simulink model "TVModel_Simulation_21"  (R2021b)
settings: Solver=FixedStepDiscrete  StartTime=0.0  StopTime=250  FixedStep=0.02  MaxStep=0.01  RelTol=1e-3
undefined symbols (not defined in the file or in its folder): MB, TV, TV_OLD
libraries: simulink x22, simulink_extras x14, eeGeneralControl x13, slpidlib x8, fuzblock x4, controlLib x4, cstblocks x3, dspstat3 x2, eeSlidingModeController x1, sharedTrackingLibrary x1
(part 8 of 9)

== matlab function TVModel_Simulation_21/Subsystem/Subsystem1/Slip Control/Traction Control/ABS/Mu Linearization ==
  data: kappa input; mu0 output; mu1 output; Fz input; a0 output
function [mu0,mu1,a0] = fcn(kappa,Fz)

LMUX = 0.93;
J_wheel = 2e5/1e6;
rs = 0.235;
m = 270/4;
tau = 13.5;
dt = 0.02;

deltaKappa = 0.01;
kappa_plus = kappa + deltaKappa;

mu0 = muX(kappa,Fz,LMUX);
mu1 = (muX(kappa_plus,Fz,LMUX)-mu0)./(deltaKappa);

a0 = Fz./vx*mu1( (1-kappa)/m + rs^2/J_wheel );

end
function mu = muX(kappa,Fz,LMUX)
    mu = ((Fz.^2.*LMUX)./1.0e+4-Fz.*LMUX.*sin(atan((Fz.*5.946e-5-6.5736e-1).*(sign(Fz.*(-1.5696e-6)+kappa+6.665e-4).*5.242e-1+1.0).*(atan((Fz.*exp(Fz.*(-1.3455e-5)+1.3455e-2).*(Fz.*(3.0./2.0e+2)+6.77e+2./1.0e+1).*(Fz.*(-1.5696e-6)+kappa+6.665e-4).*(3.33e+2./4.0e+2))./(Fz.*LMUX.*2.5847808+1.0./1.0e+2))-(Fz.*exp(Fz.*(-1.3455e-5)+1.3455e-2).*(Fz.*(3.0./2.0e+2)+6.77e+2./1.0e+1).*(Fz.*(-1.5696e-6)+kappa+6.665e-4).*(3.33e+2./4.0e+2))./(Fz.*LMUX.*2.5847808+1.0./1.0e+2))-(Fz.*exp(Fz.*(-1.3455e-5)+1.3455e-2).*(Fz.*(3.0./2.0e+2)+6.77e+2./1.0e+1).*(Fz.*(-1.5696e-6)+kappa+6.665e-4).*(3.33e+2./4.0e+2))./(Fz.*LMUX.*2.5847808+1.0./1.0e+2)).*(1.68e+2./1.25e+2)).*1.9232)./Fz;
end

== stateflow chart TVModel_Simulation_21/Subsystem/Subsystem1/Slip Control/Traction Control/ABS/Subsystem/Chart ==
  state OFF
    en,du:
    TC_max = [21];
  state ON
    en,du:
    TC_max = T_ff ;
  state SWITCHING_FILTER
    en,du:
    TC_max = TC_filter_tau*TC_max;
  (default) -> OFF
  OFF -> ON : [epsilon == 1]
  SWITCHING_FILTER -> ON [order 2] : [ epsilon == 1]
  SWITCHING_FILTER -> OFF [order 1] : [count(in(SWITCHING_FILTER)) > TC_filter_time/ts]
  ON -> SWITCHING_FILTER : [epsilon == 0]
  data: T_ff input; TC_max output; ts constant double =TV.MPC.T; TC_filter_time constant double =TV.MPC.mz_filter_time; TC_filter_tau constant double =TV.MPC.mz_filter_tau; epsilon input

== matlab function TVModel_Simulation_21/Subsystem/Subsystem1/Torque Distribution/MPC/Useful Calculations/MATLAB Function2 ==
  data: omega input; y output; t input
function y = fcn(omega,t)

omega_FL = omega(1);
omega_FR = omega(2);
omega_RL = omega(3);
omega_RR = omega(4);

T_FL = t(1);
T_FR = t(2);
T_RL = t(3);
T_RR = t(4);

eta_FL = efficiency(omega_FL,T_FL) ;
eta_FR = efficiency(omega_FR,T_FR) ;
eta_RL = efficiency(omega_RL,T_RL) ;
eta_RR = efficiency(omega_RR,T_RR) ;

y = (omega_FL*T_FL/eta_FL + omega_FR*T_FR/eta_FR + omega_RL*T_RL/eta_RL + omega_RR*T_RR/eta_RR);

end

function eta = efficiency(Omega,T)

x = T;
y = Omega; % Omega rad/s to motor

p00 =      0.7189;
p10 =     0.06443;
p01 =   0.0001287;
p20 =     -0.0128;
p11 =   9.544e-05;
p02 =  -8.738e-07;
p30 =   0.0009902;
p21 =  -6.784e-06;
p12 =  -2.146e-08;
p03 =   8.018e-10;
p40 =  -3.737e-05;
p31 =   3.242e-07;
p22 =  -4.019e-10;
p13 =   9.786e-12;
p04 =   -3.44e-13;
p50 =   5.334e-07;
p41 =  -5.236e-09;
p32 =  -4.411e-14;
p23 =   1.035e-13;
p14 =  -1.745e-15;
p05 =   5.581e-17;

eta = p00 + p10*x + p01*y + p20*x^2 + p11*x*y + p02*y^2 + p30*x^3 + p21*x^2*y ...
      + p12*x*y^2 + p03*y^3 + p40*x^4 + p31*x^3*y + p22*x^2*y^2 ...
      + p13*x*y^3 + p04*y^4 + p50*x^5 + p41*x^4*y + p32*x^3*y^2 ...
      + p23*x^2*y^3 + p14*x*y^4 + p05*y^5;

end

== stateflow chart TVModel_Simulation_21/Subsystem/Subsystem1/Slip Control/Traction Control/Slip Control/ABS/Activation logic ==
  state TS_ON
    state ABS_OFF
      en,du:
      T_min(1:4) = -T_limit(1:4);
    state ABS_ON
      state FL [parallel]
        settings: executionOrder=1
        state ABS_ACTIVE
          en:
          T_min(1) = T_actual(1);
          du:
          T_min(1) = Tmin_PI(1);
        state ABS_INACTIVE
          en,du:
          T_min(1) = -T_limit(1);
        (default) -> TS_ON.ABS_ON.FL.ABS_INACTIVE
        TS_ON.ABS_ON.FL.ABS_INACTIVE -> TS_ON.ABS_ON.FL.ABS_ACTIVE : [eps(1) <= (epsTarget(1) - slipNoise) && T_actual(1)<0]
        TS_ON.ABS_ON.FL.ABS_ACTIVE -> TS_ON.ABS_ON.FL.ABS_INACTIVE : [T_actual(1) > slipDeactPerc*Tmin_old(1)]
      state FR [parallel]
        settings: executionOrder=2
        state ABS_ACTIVE
          en:
          T_min(2) = T_actual(2);
          du:
          T_min(2) = Tmin_PI(2);
        state ABS_INACTIVE
          en,du:
          T_min(2) = -T_limit(2);
        (default) -> TS_ON.ABS_ON.FR.ABS_INACTIVE
        TS_ON.ABS_ON.FR.ABS_INACTIVE -> TS_ON.ABS_ON.FR.ABS_ACTIVE : [eps(2) <= (epsTarget(2) - slipNoise) && T_actual(2)<0]
        TS_ON.ABS_ON.FR.ABS_ACTIVE -> TS_ON.ABS_ON.FR.ABS_INACTIVE : [T_actual(2) > slipDeactPerc*Tmin_old(2) ]
      state RL [parallel]
        settings: executionOrder=3
        state ABS_ACTIVE
          en:
          T_min(3) = T_actual(3);
          du:
          T_min(3) = Tmin_PI(3);
        state ABS_INACTIVE
          en,du:
          T_min(3) = -T_limit(3);
        (default) -> TS_ON.ABS_ON.RL.ABS_INACTIVE
        TS_ON.ABS_ON.RL.ABS_INACTIVE -> TS_ON.ABS_ON.RL.ABS_ACTIVE : [eps(3) <= (epsTarget(3) - slipNoise) && T_actual(3)<0]
        TS_ON.ABS_ON.RL.ABS_ACTIVE -> TS_ON.ABS_ON.RL.ABS_INACTIVE : [T_actual(3) > slipDeactPerc*Tmin_old(3)]
      state RR [parallel]
        settings: executionOrder=4
        state ABS_ACTIVE
          en:
          T_min(4) = T_actual(4);
          du:
          T_min(4) = Tmin_PI(4);
        state ABS_INACTIVE
          en,du:
          T_min(4) = -T_limit(4);
        (default) -> TS_ON.ABS_ON.RR.ABS_INACTIVE
        TS_ON.ABS_ON.RR.ABS_INACTIVE -> TS_ON.ABS_ON.RR.ABS_ACTIVE : [eps(4) <= (epsTarget(4) - slipNoise) && T_actual(4)<0]
        TS_ON.ABS_ON.RR.ABS_ACTIVE -> TS_ON.ABS_ON.RR.ABS_INACTIVE : [T_actual(4) > slipDeactPerc*Tmin_old(4)]
    (default) -> ABS_OFF
    ABS_ON -> ABS_OFF : [TC_flag == 0]
    ABS_OFF -> ABS_ON : [TC_flag == 1]
  state TS_OFF
    en:
    T_min(1:4) =zeros(4,1);
  (default) -> TS_OFF
  TS_OFF -> TS_ON : [RTD_flag == 1]
  TS_ON -> TS_OFF : [RTD_flag == 0]
  data: Tmin_PI input size=4; epsTarget input size=4; eps input size=4; T_actual input size=4 =zeros(4,1); T_min output size=4 =zeros(4,1); T_limit input size=4; TC_flag input size=1; Tmin_old input size=4; slipNoise input double =LV.SLIP.; slipDeactPerc input; RTD_flag input

== matlab function TVModel_Simulation_21/Subsystem/Subsystem1/Slip Control/Traction Control/Slip Control/Slip computation/MATLAB Function2 ==
  data: Vx input; V_FL output; Vy input; phi_dot input; delta_L input; V_FR output; V_RL output; V_RR output; alpha_FL output; alpha_FR output; alpha_RL output; alpha_RR output; delta_R input; a input; b input; t input; Vx_min input
function [V_FL,V_FR,V_RL,V_RR,alpha_FL,alpha_FR,alpha_RL,alpha_RR]= fcn(Vx,Vy,phi_dot, delta_L,delta_R,a,b,t,Vx_min)
   
    vx_max_den = max(Vx,Vx_min);

    V_FL = (Vx-(t/2)*phi_dot)*cos(delta_L)+(Vy+a*phi_dot)*sin(delta_L);
    alpha_FL = atan((Vy+a*phi_dot)/(vx_max_den -(t/2)*phi_dot))-delta_L;

    V_FR = (Vx+(t/2)*phi_dot)*cos(delta_R)+(Vy+a*phi_dot)*sin(delta_R);
    alpha_FR = atan((Vy+a*phi_dot)/(vx_max_den + (t/2)*phi_dot))-delta_R;

    V_RL = (((Vx-(t/2)*phi_dot)^2)+((Vy-b*phi_dot)^2))^(1/2);
    alpha_RL = atan((Vy-b*phi_dot)/(vx_max_den -(t/2)*phi_dot));

    V_RR = (((Vx+(t/2)*phi_dot)^2)+((Vy-b*phi_dot)^2))^(1/2);
    alpha_RR = atan((Vy-b*phi_dot)/(vx_max_den + (t/2)*phi_dot));
         
end

== stateflow chart TVModel_Simulation_21/Subsystem/Subsystem1/Slip Control/Traction Control/Slip Control/TC/Activation logic ==
  state TS_ON
    state TC_OFF
      en:TC_Active=uint8(ones(4,1));
      en,du:
      T_max(1:4) = T_limit(1:4);
    state TC_ON
      state FL [parallel]
        settings: executionOrder=1
        state TC_ACTIVE
          en:
          TC_Active(1)=uint8(2);
          T_max(1) = abs(T_actual(1));
          du:
          T_max(1) = Tmax_PI(1);
        state TC_INACTIVE
          en:
          TC_Active(1)=uint8(1);
          T_max(1) = T_limit(1);
          du:
          T_max(1) = T_limit(1);
        (default) -> TS_ON.TC_ON.FL.TC_INACTIVE
        TS_ON.TC_ON.FL.TC_INACTIVE -> TS_ON.TC_ON.FL.TC_ACTIVE : [eps(1) >= epsTarget(1) + slipNoise]
        TS_ON.TC_ON.FL.TC_ACTIVE -> TS_ON.TC_ON.FL.TC_INACTIVE : [T_actual(1) < slipDeactPerc*Tmax_old(1)]
      state FR [parallel]
        settings: executionOrder=2
        state TC_ACTIVE
          en:
          TC_Active(2)=uint8(2);
          T_max(2) = abs(T_actual(2));
          du:
          T_max(2) = Tmax_PI(2);
        state TC_INACTIVE
          en:
          TC_Active(2)=uint8(1);
          T_max(2) = T_limit(2);
          du:
          T_max(2) = T_limit(2);
        (default) -> TS_ON.TC_ON.FR.TC_INACTIVE
        TS_ON.TC_ON.FR.TC_INACTIVE -> TS_ON.TC_ON.FR.TC_ACTIVE : [eps(2) >= epsTarget(2) + slipNoise]
        TS_ON.TC_ON.FR.TC_ACTIVE -> TS_ON.TC_ON.FR.TC_INACTIVE : [T_actual(2) < slipDeactPerc*Tmax_old(2) ]
      state RL [parallel]
        settings: executionOrder=3
        state TC_ACTIVE
          en:
          TC_Active(3)=uint8(2);
          T_max(3) = abs(T_actual(3));
          du:
          T_max(3) = Tmax_PI(3);
        state TC_INACTIVE
          en:
          TC_Active(3)=uint8(1);
          T_max(3) = T_limit(3);
          du:
          T_max(3) = T_limit(3);
        (default) -> TS_ON.TC_ON.RL.TC_INACTIVE
        TS_ON.TC_ON.RL.TC_INACTIVE -> TS_ON.TC_ON.RL.TC_ACTIVE : [eps(3) >= epsTarget(3) + slipNoise]
        TS_ON.TC_ON.RL.TC_ACTIVE -> TS_ON.TC_ON.RL.TC_INACTIVE : [T_actual(3) < slipDeactPerc*Tmax_old(3)]
      state RR [parallel]
        settings: executionOrder=4
        state TC_ACTIVE
          en:
          TC_Active(4)=uint8(2);
          T_max(4) = abs(T_actual(4));
          du:
          T_max(4) = Tmax_PI(4);
        state TC_INACTIVE
          en:
          TC_Active(4)=uint8(1);
          T_max(4) = T_limit(4);
          du:
          T_max(4) = T_limit(4);
        (default) -> TS_ON.TC_ON.RR.TC_INACTIVE
        TS_ON.TC_ON.RR.TC_INACTIVE -> TS_ON.TC_ON.RR.TC_ACTIVE : [eps(4) >= epsTarget(4) + slipNoise]
        TS_ON.TC_ON.RR.TC_ACTIVE -> TS_ON.TC_ON.RR.TC_INACTIVE : [T_actual(4) < slipDeactPerc*Tmax_old(4)]
    (default) -> TC_OFF
    TC_ON -> TC_OFF : [TC_flag == 0]
    TC_OFF -> TC_ON : [TC_flag == 1]
  state TS_OFF
    en:
    T_max(1:4) = zeros(4,1);
  (default) -> TS_OFF
  TS_OFF -> TS_ON : [RTD_flag == 1]
  TS_ON -> TS_OFF : [RTD_flag == 0]
  data: Tmax_PI input size=4; epsTarget input size=4; eps input size=4; T_actual input size=4 =zeros(4,1); T_max output size=4 =zeros(4,1); T_limit input size=4; TC_flag input size=1; Tmax_old input size=4; slipNoise input double =LV.slipNoise; slipDeactPerc input; RTD_flag input; TC_Active output uint8 size=4

== matlab function TVModel_Simulation_21/Subsystem/Subsystem1/Slip Control/Traction Control/Slip Control/slip ratio/MATLAB Function ==
  data: vx_wheels input size=4; k output size=4; wR input size=4; vx_min input
function k = slipRatio(vx_wheels,wR,vx_min)

k = zeros(4,1);

for i = 1:4
   k(i) = (wR(i) - vx_wheels(i))/max([vx_wheels(i), wR(i), vx_min]);
end

end

== matlab function TVModel_Simulation_21/Subsystem/Subsystem1/Torque Distribution/MPC/Mz Generation/MATLAB Function3 ==
  data: ubx input; lbx input; Mzlim output; delta input
function Mzlim = fcn(ubx,lbx,delta)
tf = 1.27;
tr = 1.27;
a = 0.765;

delta_l = delta(1);
delta_r = delta(2);

T_FL_max = ubx(1);
T_FR_min = lbx(2);
T_RL_max = ubx(3);
T_RR_min = lbx(4);

Mzlim = +(a.*sin(delta_l)-tf/2.*cos(delta_l))*T_FL_max +(a.*sin(delta_r)+tf/2*cos(delta_r))*T_FR_min -tr/2*T_RL_max +tr/2*T_RR_min;

== matlab function TVModel_Simulation_21/Subsystem/Subsystem1/Torque Distribution/MPC/Mz Generation/MATLAB Function4 ==
  data: ubx input; lbx input; Mzlim output; delta input
function Mzlim = fcn(ubx,lbx,delta)
tf = 1.27;
tr = 1.27;
a = 0.765;

delta_l = delta(1);
delta_r = delta(2);

T_FL_min = lbx(1);
T_FR_max = ubx(2);
T_RL_min = lbx(3);
T_RR_max = ubx(4);

Mzlim = +(a.*sin(delta_l)-tf/2.*cos(delta_l))*T_FL_min +(a.*sin(delta_r)+tf/2*cos(delta_r))*T_FR_max -tr/2*T_RL_min +tr/2*T_RR_max;

== matlab function TVModel_Simulation_21/Subsystem/Subsystem1/Torque Distribution/MPC/Useful Calculations/MATLAB Function1 ==
  data: u input; deltag3 output; deltag4 output
function [deltag3,deltag4] = fcn(u)

deltag3 = u(2) - u(4);
deltag4 = u(1) - u(3);

== matlab function TVModel_Simulation_21/Subsystem/Subsystem1/Slip Control/Traction Control/TC/MATLAB Function ==
  data: u_max_old input; vx input; u output; Fz input; kappa input
function u = linear_mpc(u_max_old,vx,Fz,kappa)

LMU = 0.8;
rs = 0.235;
Iw = 2e5/1e6;
dt = 0.2;
tau = 13.5;
dt = 0.02;
g = 9.81;

B = rs^2/Iw/vx*dt;

u = zeros(4,1);
u(1) = tc(u_max_old(1),vx,Fz(1),kappa(1));
u(2) = tc(u_max_old(2),vx,Fz(2),kappa(2));
u(3) = tc(u_max_old(3),vx,Fz(3),kappa(3));
u(4) = tc(u_max_old(4),vx,Fz(4),kappa(4));

end
% Astar = (0.0148*cos(0.989*atan((atan(0.159/(635.0*kappa^2 + 1.0)^(1/2)) - 0.159/(635.0*kappa^2 + 1.0)^(1/2))*(2.08e-4*Fz + 0.117) - 0.159/(635.0*kappa^2 + 1.0)^(1/2)))*(1.0e-4*Fz^2*LMU - 1.92*Fz*LMU*sin(1.41*atan((4.17e-5*Fz - 0.46)*(0.524*sign(kappa - 1.57e-6*Fz + 6.66e-4) + 1.0)*(atan((0.7*Fz*exp(0.0135 - 1.35e-5*Fz)*(0.015*Fz + 67.7)*(kappa - 1.57e-6*Fz + 6.66e-4))/(2.71*Fz*LMU + 0.01)) - (0.7*Fz*exp(0.0135 - 1.35e-5*Fz)*(0.015*Fz + 67.7)*(kappa - 1.57e-6*Fz + 6.66e-4))/(2.71*Fz*LMU + 0.01)) - (0.7*Fz*exp(0.0135 - 1.35e-5*Fz)*(0.015*Fz + 67.7)*(kappa - 1.57e-6*Fz + 6.66e-4))/(2.71*Fz*LMU + 0.01)))))/(vx*cos(0.989*atan(0.159/(635.0*kappa^2 + 1.0)^(1/2) - 1.0*(atan(0.159/(635.0*kappa^2 + 1.0)^(1/2)) - 0.159/(635.0*kappa^2 + 1.0)^(1/2))*(2.08e-4*Fz + 0.117)))) + (0.989*sin(0.989*atan((atan(0.159/(635.0*kappa^2 + 1.0)^(1/2)) - 0.159/(635.0*kappa^2 + 1.0)^(1/2))*(2.08e-4*Fz + 0.117) - 0.159/(635.0*kappa^2 + 1.0)^(1/2)))*(1.0e-4*Fz^2*LMU - 1.92*Fz*LMU*sin(1.41*atan((4.17e-5*Fz - 0.46)*(0.524*sign(kappa - 1.57e-6*Fz + 6.66e-4) + 1.0)*(atan((0.7*Fz*exp(0.0135 - 1.35e-5*Fz)*(0.015*Fz + 67.7)*(kappa - 1.57e-6*Fz + 6.66e-4))/(2.71*Fz*LMU + 0.01)) - (0.7*Fz*exp(0.0135 - 1.35e-5*Fz)*(0.015*Fz + 67.7)*(kappa - 1.57e-6*Fz + 6.66e-4))/(2.71*Fz*LMU + 0.01)) - (0.7*Fz*exp(0.0135 - 1.35e-5*Fz)*(0.015*Fz + 67.7)*(kappa - 1.57e-6*Fz + 6.66e-4))/(2.71*Fz*LMU + 0.01))))*((2.08e-4*Fz + 0.117)*((101.0*kappa)/(635.0*kappa^2 + 1.0)^(3/2) - (101.0*kappa)/((635.0*kappa^2 + 1.0)^(3/2)*(0.0254/(635.0*kappa^2 + 1.0) + 1.0))) + (101.0*kappa)/(635.0*kappa^2 + 1.0)^(3/2))*(rs^2/Iw - 0.0148*kappa + 0.0148))/(vx*cos(0.989*atan(0.159/(635.0*kappa^2 + 1.0)^(1/2) - 1.0*(atan(0.159/(635.0*kappa^2 + 1.0)^(1/2)) - 0.159/(635.0*kappa^2 + 1.0)^(1/2))*(2.08e-4*Fz + 0.117)))*(((atan(0.159/(635.0*kappa^2 + 1.0)^(1/2)) - 0.159/(635.0*kappa^2 + 1.0)^(1/2))*(2.08e-4*Fz + 0.117) - 0.159/(635.0*kappa^2 + 1.0)^(1/2))^2 + 1.0)) + (0.989*cos(0.989*atan((atan(0.159/(635.0*kappa^2 + 1.0)^(1/2)) - 0.159/(635.0*kappa^2 + 1.0)^(1/2))*(2.08e-4*Fz + 0.117) - 0.159/(635.0*kappa^2 + 1.0)^(1/2)))*sin(0.989*atan(0.159/(635.0*kappa^2 + 1.0)^(1/2) - 1.0*(atan(0.159/(635.0*kappa^2 + 1.0)^(1/2)) - 0.159/(635.0*kappa^2 + 1.0)^(1/2))*(2.08e-4*Fz + 0.117)))*(1.0e-4*Fz^2*LMU - 1.92*Fz*LMU*sin(1.41*atan((4.17e-5*Fz - 0.46)*(0.524*sign(kappa - 1.57e-6*Fz + 6.66e-4) + 1.0)*(atan((0.7*Fz*exp(0.0135 - 1.35e-5*Fz)*(0.015*Fz + 67.7)*(kappa - 1.57e-6*Fz + 6.66e-4))/(2.71*Fz*LMU + 0.01)) - (0.7*Fz*exp(0.0135 - 1.35e-5*Fz)*(0.015*Fz + 67.7)*(kappa - 1.57e-6*Fz + 6.66e-4))/(2.71*Fz*LMU + 0.01)) - (0.7*Fz*exp(0.0135 - 1.35e-5*Fz)*(0.015*Fz + 67.7)*(kappa - 1.57e-6*Fz + 6.66e-4))/(2.71*Fz*LMU + 0.01))))*((2.08e-4*Fz + 0.117)*((101.0*kappa)/(635.0*kappa^2 + 1.0)^(3/2) - (101.0*kappa)/((635.0*kappa^2 + 1.0)^(3/2)*(0.0253/(635.0*kappa^2 + 1.0) + 1.0))) + (101.0*kappa)/(635.0*kappa^2 + 1.0)^(3/2))*(rs^2/Iw - 0.0148*kappa + 0.0148))/(vx*cos(0.989*atan(0.159/(635.0*kappa^2 + 1.0)^(1/2) - 1.0*(atan(0.159/(635.0*kappa^2 + 1.0)^(1/2)) - 0.159/(635.0*kappa^2 + 1.0)^(1/2))*(2.08e-4*Fz + 0.117)))^2*((1.0*(atan(0.159/(635.0*kappa^2 + 1.0)^(1/2)) - 0.159/(635.0*kappa^2 + 1.0)^(1/2))*(2.08e-4*Fz + 0.117) - 0.159/(635.0*kappa^2 + 1.0)^(1/2))^2 + 1.0)) - (2.71*Fz*LMU*cos(1.41*atan((4.17e-5*Fz - 0.46)*(0.524*sign(kappa - 1.57e-6*Fz + 6.66e-4) + 1.0)*(atan((0.7*Fz*exp(0.0135 - 1.35e-5*Fz)*(0.015*Fz + 67.7)*(kappa - 1.57e-6*Fz + 6.66e-4))/(2.71*Fz*LMU + 0.01)) - (0.7*Fz*exp(0.0135 - 1.35e-5*Fz)*(0.015*Fz + 67.7)*(kappa - 1.57e-6*Fz + 6.66e-4))/(2.71*Fz*LMU + 0.01)) - (0.7*Fz*exp(0.0135 - 1.35e-5*Fz)*(0.015*Fz + 67.7)*(kappa - 1.57e-6*Fz + 6.66e-4))/(2.71*Fz*LMU + 0.01)))*cos(0.989*atan((atan(0.159/(635.0*kappa^2 + 1.0)^(1/2)) - 0.159/(635.0*kappa^2 + 1.0)^(1/2))*(2.08e-4*Fz + 0.117) - 0.159/(635.0*kappa^2 + 1.0)^(1/2)))*(((0.7*Fz*exp(0.0135 - 1.35e-5*Fz)*(0.015*Fz + 67.7))/(2.71*Fz*LMU + 0.01) - (0.7*Fz*exp(0.0135 - 1.35e-5*Fz)*(0.015*Fz + 67.7))/(((0.49*Fz^2*exp(0.027 - 2.7e-5*Fz)*(0.015*Fz + 67.7)^2*(kappa - 1.57e-6*Fz + 6.66e-4)^2)/(2.71*Fz*LMU + 0.01)^2 + 1.0)*(2.71*Fz*LMU + 0.01)))*(4.17e-5*Fz - 0.46)*(0.524*sign(kappa - 1.57e-6*Fz + 6.66e-4) + 1.0) - 1.05*dirac(kappa - 1.57e-6*Fz + 6.66e-4)*(4.17e-5*Fz - 0.46)*(atan((0.7*Fz*exp(0.0135 - 1.35e-5*Fz)*(0.015*Fz + 67.7)*(kappa - 1.57e-6*Fz + 6.66e-4))/(2.71*Fz*LMU + 0.01)) - (0.7*Fz*exp(0.0135 - 1.35e-5*Fz)*(0.015*Fz + 67.7)*(kappa - 1.57e-6*Fz + 6.66e-4))/(2.71*Fz*LMU + 0.01)) + (0.7*Fz*exp(0.0135 - 1.35e-5*Fz)*(0.015*Fz + 67.7))/(2.71*Fz*LMU + 0.01))*(rs^2/Iw - 0.0148*kappa + 0.0148))/(vx*cos(0.989*atan(0.159/(635.0*kappa^2 + 1.0)^(1/2) - 1.0*(atan(0.159/(635.0*kappa^2 + 1.0)^(1/2)) - 0.159/(635.0*kappa^2 + 1.0)^(1/2))*(2.08e-4*Fz + 0.117)))*(((4.17e-5*Fz - 0.46)*(0.524*sign(kappa - 1.57e-6*Fz + 6.66e-4) + 1.0)*(atan((0.7*Fz*exp(0.0135 - 1.35e-5*Fz)*(0.015*Fz + 67.7)*(kappa - 1.57e-6*Fz + 6.66e-4))/(2.71*Fz*LMU + 0.01)) - (0.7*Fz*exp(0.0135 - 1.35e-5*Fz)*(0.015*Fz + 67.7)*(kappa - 1.57e-6*Fz + 6.66e-4))/(2.71*Fz*LMU + 0.01)) - (0.7*Fz*exp(0.0135 - 1.35e-5*Fz)*(0.015*Fz + 67.7)*(kappa - 1.57e-6*Fz + 6.66e-4))/(2.71*Fz*LMU + 0.01))^2 + 1.0))
function u_ij = tc(u_max_old,vx,Fz,kappa)
fx = -(1.0*cos(0.989*atan((atan(0.159/(635.0*kappa^2 + 1.0)^(1/2)) - 0.159/(635.0*kappa^2 + 1.0)^(1/2))*(2.08e-4*Fz + 0.117) - 0.159/(635.0*kappa^2 + 1.0)^(1/2)))*(1.0e-4*Fz^2*LMU - 1.92*Fz*LMU*sin(1.41*atan((4.17e-5*Fz - 0.46)*(0.524*sign(kappa - 1.57e-6*Fz + 6.66e-4) + 1.0)*(atan((0.7*Fz*exp(0.0135 - 1.35e-5*Fz)*(0.015*Fz + 67.7)*(kappa - 1.57e-6*Fz + 6.66e-4))/(2.71*Fz*LMU + 0.01)) - (0.7*Fz*exp(0.0135 - 1.35e-5*Fz)*(0.015*Fz + 67.7)*(kappa - 1.57e-6*Fz + 6.66e-4))/(2.71*Fz*LMU + 0.01)) - (0.7*Fz*exp(0.0135 - 1.35e-5*Fz)*(0.015*Fz + 67.7)*(kappa - 1.57e-6*Fz + 6.66e-4))/(2.71*Fz*LMU + 0.01))))*(rs^2/Iw - 0.0148*kappa + 0.0148))/(vx*cos(0.989*atan((atan(0.159/(635.0*kappa^2 + 1.0)^(1/2)) - 0.159/(635.0*kappa^2 + 1.0)^(1/2))*(2.08e-4*Fz + 0.117) - 0.159/(635.0*kappa^2 + 1.0)^(1/2))));
delta_kappa = 0.001;
kappa_plus = kappa + delta_kappa;
fx_plus = -(1.0*cos(0.989*atan((atan(0.159/(635.0*kappa_plus^2 + 1.0)^(1/2)) - 0.159/(635.0*kappa_plus^2 + 1.0)^(1/2))*(2.08e-4*Fz + 0.117) - 0.159/(635.0*kappa_plus^2 + 1.0)^(1/2)))*(1.0e-4*Fz^2*LMU - 1.92*Fz*LMU*sin(1.41*atan((4.17e-5*Fz - 0.46)*(0.524*sign(kappa_plus - 1.57e-6*Fz + 6.66e-4) + 1.0)*(atan((0.7*Fz*exp(0.0135 - 1.35e-5*Fz)*(0.015*Fz + 67.7)*(kappa_plus - 1.57e-6*Fz + 6.66e-4))/(2.71*Fz*LMU + 0.01)) - (0.7*Fz*exp(0.0135 - 1.35e-5*Fz)*(0.015*Fz + 67.7)*(kappa_plus - 1.57e-6*Fz + 6.66e-4))/(2.71*Fz*LMU + 0.01)) - (0.7*Fz*exp(0.0135 - 1.35e-5*Fz)*(0.015*Fz + 67.7)*(kappa_plus - 1.57e-6*Fz + 6.66e-4))/(2.71*Fz*LMU + 0.01))))*(rs^2/Iw - 0.0148*kappa_plus + 0.0148))/(vx*cos(0.989*atan((atan(0.159/(635.0*kappa_plus^2 + 1.0)^(1/2)) - 0.159/(635.0*kappa_plus^2 + 1.0)^(1/2))*(2.08e-4*Fz + 0.117) - 0.159/(635.0*kappa_plus^2 + 1.0)^(1/2))));

Astar = (fx_plus - fx)/delta_kappa;

A = (1 + Astar*dt);

% ~~~~~~~~~~~~~~~~~~~~~~~~~~~~~~~~~~~~~~~~~~~~~~~~~~~~~~~~~~~~~~~~~~~~~~~ %
kappa_ref = 0.1;

% Q = 1e6;
Q = 5e5;
R = 0e-5;

u_ij = u_max_old + (B*Q*B + R)*( (Q*B)*kappa_ref - (A*Q*B)*kappa )/tau;
end

== matlab function TVModel_Simulation_21/Subsystem/Subsystem1/Slip Control/Traction Control/Subsystem2/MATLAB Function1 ==
  data: u_max_old input; vx input; u output; Fz input; kappa input
function u = linear_mpc(u_max_old,vx,Fz,kappa)

% Astar = (0.0148*cos(0.989*atan((atan(0.159/(635.0*kappa^2 + 1.0)^(1/2)) - 0.159/(635.0*kappa^2 + 1.0)^(1/2))*(2.08e-4*Fz + 0.117) - 0.159/(635.0*kappa^2 + 1.0)^(1/2)))*(1.0e-4*Fz^2*LMU - 1.92*Fz*LMU*sin(1.41*atan((4.17e-5*Fz - 0.46)*(0.524*sign(kappa - 1.57e-6*Fz + 6.66e-4) + 1.0)*(atan((0.7*Fz*exp(0.0135 - 1.35e-5*Fz)*(0.015*Fz + 67.7)*(kappa - 1.57e-6*Fz + 6.66e-4))/(2.71*Fz*LMU + 0.01)) - (0.7*Fz*exp(0.0135 - 1.35e-5*Fz)*(0.015*Fz + 67.7)*(kappa - 1.57e-6*Fz + 6.66e-4))/(2.71*Fz*LMU + 0.01)) - (0.7*Fz*exp(0.0135 - 1.35e-5*Fz)*(0.015*Fz + 67.7)*(kappa - 1.57e-6*Fz + 6.66e-4))/(2.71*Fz*LMU + 0.01)))))/(vx*cos(0.989*atan(0.159/(635.0*kappa^2 + 1.0)^(1/2) - 1.0*(atan(0.159/(635.0*kappa^2 + 1.0)^(1/2)) - 0.159/(635.0*kappa^2 + 1.0)^(1/2))*(2.08e-4*Fz + 0.117)))) + (0.989*sin(0.989*atan((atan(0.159/(635.0*kappa^2 + 1.0)^(1/2)) - 0.159/(635.0*kappa^2 + 1.0)^(1/2))*(2.08e-4*Fz + 0.117) - 0.159/(635.0*kappa^2 + 1.0)^(1/2)))*(1.0e-4*Fz^2*LMU - 1.92*Fz*LMU*sin(1.41*atan((4.17e-5*Fz - 0.46)*(0.524*sign(kappa - 1.57e-6*Fz + 6.66e-4) + 1.0)*(atan((0.7*Fz*exp(0.0135 - 1.35e-5*Fz)*(0.015*Fz + 67.7)*(kappa - 1.57e-6*Fz + 6.66e-4))/(2.71*Fz*LMU + 0.01)) - (0.7*Fz*exp(0.0135 - 1.35e-5*Fz)*(0.015*Fz + 67.7)*(kappa - 1.57e-6*Fz + 6.66e-4))/(2.71*Fz*LMU + 0.01)) - (0.7*Fz*exp(0.0135 - 1.35e-5*Fz)*(0.015*Fz + 67.7)*(kappa - 1.57e-6*Fz + 6.66e-4))/(2.71*Fz*LMU + 0.01))))*((2.08e-4*Fz + 0.117)*((101.0*kappa)/(635.0*kappa^2 + 1.0)^(3/2) - (101.0*kappa)/((635.0*kappa^2 + 1.0)^(3/2)*(0.0254/(635.0*kappa^2 + 1.0) + 1.0))) + (101.0*kappa)/(635.0*kappa^2 + 1.0)^(3/2))*(rs^2/Iw - 0.0148*kappa + 0.0148))/(vx*cos(0.989*atan(0.159/(635.0*kappa^2 + 1.0)^(1/2) - 1.0*(atan(0.159/(635.0*kappa^2 + 1.0)^(1/2)) - 0.159/(635.0*kappa^2 + 1.0)^(1/2))*(2.08e-4*Fz + 0.117)))*(((atan(0.159/(635.0*kappa^2 + 1.0)^(1/2)) - 0.159/(635.0*kappa^2 + 1.0)^(1/2))*(2.08e-4*Fz + 0.117) - 0.159/(635.0*kappa^2 + 1.0)^(1/2))^2 + 1.0)) + (0.989*cos(0.989*atan((atan(0.159/(635.0*kappa^2 + 1.0)^(1/2)) - 0.159/(635.0*kappa^2 + 1.0)^(1/2))*(2.08e-4*Fz + 0.117) - 0.159/(635.0*kappa^2 + 1.0)^(1/2)))*sin(0.989*atan(0.159/(635.0*kappa^2 + 1.0)^(1/2) - 1.0*(atan(0.159/(635.0*kappa^2 + 1.0)^(1/2)) - 0.159/(635.0*kappa^2 + 1.0)^(1/2))*(2.08e-4*Fz + 0.117)))*(1.0e-4*Fz^2*LMU - 1.92*Fz*LMU*sin(1.41*atan((4.17e-5*Fz - 0.46)*(0.524*sign(kappa - 1.57e-6*Fz + 6.66e-4) + 1.0)*(atan((0.7*Fz*exp(0.0135 - 1.35e-5*Fz)*(0.015*Fz + 67.7)*(kappa - 1.57e-6*Fz + 6.66e-4))/(2.71*Fz*LMU + 0.01)) - (0.7*Fz*exp(0.0135 - 1.35e-5*Fz)*(0.015*Fz + 67.7)*(kappa - 1.57e-6*Fz + 6.66e-4))/(2.71*Fz*LMU + 0.01)) - (0.7*Fz*exp(0.0135 - 1.35e-5*Fz)*(0.015*Fz + 67.7)*(kappa - 1.57e-6*Fz + 6.66e-4))/(2.71*Fz*LMU + 0.01))))*((2.08e-4*Fz + 0.117)*((101.0*kappa)/(635.0*kappa^2 + 1.0)^(3/2) - (101.0*kappa)/((635.0*kappa^2 + 1.0)^(3/2)*(0.0253/(635.0*kappa^2 + 1.0) + 1.0))) + (101.0*kappa)/(635.0*kappa^2 + 1.0)^(3/2))*(rs^2/Iw - 0.0148*kappa + 0.0148))/(vx*cos(0.989*atan(0.159/(635.0*kappa^2 + 1.0)^(1/2) - 1.0*(atan(0.159/(635.0*kappa^2 + 1.0)^(1/2)) - 0.159/(635.0*kappa^2 + 1.0)^(1/2))*(2.08e-4*Fz + 0.117)))^2*((1.0*(atan(0.159/(635.0*kappa^2 + 1.0)^(1/2)) - 0.159/(635.0*kappa^2 + 1.0)^(1/2))*(2.08e-4*Fz + 0.117) - 0.159/(635.0*kappa^2 + 1.0)^(1/2))^2 + 1.0)) - (2.71*Fz*LMU*cos(1.41*atan((4.17e-5*Fz - 0.46)*(0.524*sign(kappa - 1.57e-6*Fz + 6.66e-4) + 1.0)*(atan((0.7*Fz*exp(0.0135 - 1.35e-5*Fz)*(0.015*Fz + 67.7)*(kappa - 1.57e-6*Fz + 6.66e-4))/(2.71*Fz*LMU + 0.01)) - (0.7*Fz*exp(0.0135 - 1.35e-5*Fz)*(0.015*Fz + 67.7)*(kappa - 1.57e-6*Fz + 6.66e-4))/(2.71*Fz*LMU + 0.01)) - (0.7*Fz*exp(0.0135 - 1.35e-5*Fz)*(0.015*Fz + 67.7)*(kappa - 1.57e-6*Fz + 6.66e-4))/(2.71*Fz*LMU + 0.01)))*cos(0.989*atan((atan(0.159/(635.0*kappa^2 + 1.0)^(1/2)) - 0.159/(635.0*kappa^2 + 1.0)^(1/2))*(2.08e-4*Fz + 0.117) - 0.159/(635.0*kappa^2 + 1.0)^(1/2)))*(((0.7*Fz*exp(0.0135 - 1.35e-5*Fz)*(0.015*Fz + 67.7))/(2.71*Fz*LMU + 0.01) - (0.7*Fz*exp(0.0135 - 1.35e-5*Fz)*(0.015*Fz + 67.7))/(((0.49*Fz^2*exp(0.027 - 2.7e-5*Fz)*(0.015*Fz + 67.7)^2*(kappa - 1.57e-6*Fz + 6.66e-4)^2)/(2.71*Fz*LMU + 0.01)^2 + 1.0)*(2.71*Fz*LMU + 0.01)))*(4.17e-5*Fz - 0.46)*(0.524*sign(kappa - 1.57e-6*Fz + 6.66e-4) + 1.0) - 1.05*dirac(kappa - 1.57e-6*Fz + 6.66e-4)*(4.17e-5*Fz - 0.46)*(atan((0.7*Fz*exp(0.0135 - 1.35e-5*Fz)*(0.015*Fz + 67.7)*(kappa - 1.57e-6*Fz + 6.66e-4))/(2.71*Fz*LMU + 0.01)) - (0.7*Fz*exp(0.0135 - 1.35e-5*Fz)*(0.015*Fz + 67.7)*(kappa - 1.57e-6*Fz + 6.66e-4))/(2.71*Fz*LMU + 0.01)) + (0.7*Fz*exp(0.0135 - 1.35e-5*Fz)*(0.015*Fz + 67.7))/(2.71*Fz*LMU + 0.01))*(rs^2/Iw - 0.0148*kappa + 0.0148))/(vx*cos(0.989*atan(0.159/(635.0*kappa^2 + 1.0)^(1/2) - 1.0*(atan(0.159/(635.0*kappa^2 + 1.0)^(1/2)) - 0.159/(635.0*kappa^2 + 1.0)^(1/2))*(2.08e-4*Fz + 0.117)))*(((4.17e-5*Fz - 0.46)*(0.524*sign(kappa - 1.57e-6*Fz + 6.66e-4) + 1.0)*(atan((0.7*Fz*exp(0.0135 - 1.35e-5*Fz)*(0.015*Fz + 67.7)*(kappa - 1.57e-6*Fz + 6.66e-4))/(2.71*Fz*LMU + 0.01)) - (0.7*Fz*exp(0.0135 - 1.35e-5*Fz)*(0.015*Fz + 67.7)*(kappa - 1.57e-6*Fz + 6.66e-4))/(2.71*Fz*LMU + 0.01)) - (0.7*Fz*exp(0.0135 - 1.35e-5*Fz)*(0.015*Fz + 67.7)*(kappa - 1.57e-6*Fz + 6.66e-4))/(2.71*Fz*LMU + 0.01))^2 + 1.0))

LMU = 0.8;
rs = 0.235;
Iw = 2e5/1e6;
dt = 0.2;
tau = 13.5;
dt = 0.02;
g = 9.81;

B = rs^2/Iw/vx*dt;

fx = -(1.0*cos(0.989*atan((atan(0.159/(635.0*kappa^2 + 1.0)^(1/2)) - 0.159/(635.0*kappa^2 + 1.0)^(1/2))*(2.08e-4*Fz + 0.117) - 0.159/(635.0*kappa^2 + 1.0)^(1/2)))*(1.0e-4*Fz^2*LMU - 1.92*Fz*LMU*sin(1.41*atan((4.17e-5*Fz - 0.46)*(0.524*sign(kappa - 1.57e-6*Fz + 6.66e-4) + 1.0)*(atan((0.7*Fz*exp(0.0135 - 1.35e-5*Fz)*(0.015*Fz + 67.7)*(kappa - 1.57e-6*Fz + 6.66e-4))/(2.71*Fz*LMU + 0.01)) - (0.7*Fz*exp(0.0135 - 1.35e-5*Fz)*(0.015*Fz + 67.7)*(kappa - 1.57e-6*Fz + 6.66e-4))/(2.71*Fz*LMU + 0.01)) - (0.7*Fz*exp(0.0135 - 1.35e-5*Fz)*(0.015*Fz + 67.7)*(kappa - 1.57e-6*Fz + 6.66e-4))/(2.71*Fz*LMU + 0.01))))*(rs^2/Iw - 0.0148*kappa + 0.0148))/(vx*cos(0.989*atan((atan(0.159/(635.0*kappa^2 + 1.0)^(1/2)) - 0.159/(635.0*kappa^2 + 1.0)^(1/2))*(2.08e-4*Fz + 0.117) - 0.159/(635.0*kappa^2 + 1.0)^(1/2))));
delta_kappa = 0.001;
kappa_plus = kappa + delta_kappa;
fx_plus = -(1.0*cos(0.989*atan((atan(0.159/(635.0*kappa_plus^2 + 1.0)^(1/2)) - 0.159/(635.0*kappa_plus^2 + 1.0)^(1/2))*(2.08e-4*Fz + 0.117) - 0.159/(635.0*kappa_plus^2 + 1.0)^(1/2)))*(1.0e-4*Fz^2*LMU - 1.92*Fz*LMU*sin(1.41*atan((4.17e-5*Fz - 0.46)*(0.524*sign(kappa_plus - 1.57e-6*Fz + 6.66e-4) + 1.0)*(atan((0.7*Fz*exp(0.0135 - 1.35e-5*Fz)*(0.015*Fz + 67.7)*(kappa_plus - 1.57e-6*Fz + 6.66e-4))/(2.71*Fz*LMU + 0.01)) - (0.7*Fz*exp(0.0135 - 1.35e-5*Fz)*(0.015*Fz + 67.7)*(kappa_plus - 1.57e-6*Fz + 6.66e-4))/(2.71*Fz*LMU + 0.01)) - (0.7*Fz*exp(0.0135 - 1.35e-5*Fz)*(0.015*Fz + 67.7)*(kappa_plus - 1.57e-6*Fz + 6.66e-4))/(2.71*Fz*LMU + 0.01))))*(rs^2/Iw - 0.0148*kappa_plus + 0.0148))/(vx*cos(0.989*atan((atan(0.159/(635.0*kappa_plus^2 + 1.0)^(1/2)) - 0.159/(635.0*kappa_plus^2 + 1.0)^(1/2))*(2.08e-4*Fz + 0.117) - 0.159/(635.0*kappa_plus^2 + 1.0)^(1/2))));

Astar = (fx_plus - fx)/delta_kappa;

A = (1 + Astar*dt);

% ~~~~~~~~~~~~~~~~~~~~~~~~~~~~~~~~~~~~~~~~~~~~~~~~~~~~~~~~~~~~~~~~~~~~~~~ %
kappa_ref = 0.1;

% Q = 1e6;
Q = 1e3;
R = 0e-5;

u = u_max_old + (B*Q*B + R)*( (Q*B)*kappa_ref - (A*Q*B)*kappa )/tau;
end

== matlab function TVModel_Simulation_21/Subsystem/Subsystem1/Slip Control/Traction Control/Subsystem2/MATLAB Function2 ==
  data: u_max_old input; vx input; u output; Fz input; kappa input
function u = linear_mpc(u_max_old,vx,Fz,kappa)

% Astar = (0.0148*cos(0.989*atan((atan(0.159/(635.0*kappa^2 + 1.0)^(1/2)) - 0.159/(635.0*kappa^2 + 1.0)^(1/2))*(2.08e-4*Fz + 0.117) - 0.159/(635.0*kappa^2 + 1.0)^(1/2)))*(1.0e-4*Fz^2*LMU - 1.92*Fz*LMU*sin(1.41*atan((4.17e-5*Fz - 0.46)*(0.524*sign(kappa - 1.57e-6*Fz + 6.66e-4) + 1.0)*(atan((0.7*Fz*exp(0.0135 - 1.35e-5*Fz)*(0.015*Fz + 67.7)*(kappa - 1.57e-6*Fz + 6.66e-4))/(2.71*Fz*LMU + 0.01)) - (0.7*Fz*exp(0.0135 - 1.35e-5*Fz)*(0.015*Fz + 67.7)*(kappa - 1.57e-6*Fz + 6.66e-4))/(2.71*Fz*LMU + 0.01)) - (0.7*Fz*exp(0.0135 - 1.35e-5*Fz)*(0.015*Fz + 67.7)*(kappa - 1.57e-6*Fz + 6.66e-4))/(2.71*Fz*LMU + 0.01)))))/(vx*cos(0.989*atan(0.159/(635.0*kappa^2 + 1.0)^(1/2) - 1.0*(atan(0.159/(635.0*kappa^2 + 1.0)^(1/2)) - 0.159/(635.0*kappa^2 + 1.0)^(1/2))*(2.08e-4*Fz + 0.117)))) + (0.989*sin(0.989*atan((atan(0.159/(635.0*kappa^2 + 1.0)^(1/2)) - 0.159/(635.0*kappa^2 + 1.0)^(1/2))*(2.08e-4*Fz + 0.117) - 0.159/(635.0*kappa^2 + 1.0)^(1/2)))*(1.0e-4*Fz^2*LMU - 1.92*Fz*LMU*sin(1.41*atan((4.17e-5*Fz - 0.46)*(0.524*sign(kappa - 1.57e-6*Fz + 6.66e-4) + 1.0)*(atan((0.7*Fz*exp(0.0135 - 1.35e-5*Fz)*(0.015*Fz + 67.7)*(kappa - 1.57e-6*Fz + 6.66e-4))/(2.71*Fz*LMU + 0.01)) - (0.7*Fz*exp(0.0135 - 1.35e-5*Fz)*(0.015*Fz + 67.7)*(kappa - 1.57e-6*Fz + 6.66e-4))/(2.71*Fz*LMU + 0.01)) - (0.7*Fz*exp(0.0135 - 1.35e-5*Fz)*(0.015*Fz + 67.7)*(kappa - 1.57e-6*Fz + 6.66e-4))/(2.71*Fz*LMU + 0.01))))*((2.08e-4*Fz + 0.117)*((101.0*kappa)/(635.0*kappa^2 + 1.0)^(3/2) - (101.0*kappa)/((635.0*kappa^2 + 1.0)^(3/2)*(0.0254/(635.0*kappa^2 + 1.0) + 1.0))) + (101.0*kappa)/(635.0*kappa^2 + 1.0)^(3/2))*(rs^2/Iw - 0.0148*kappa + 0.0148))/(vx*cos(0.989*atan(0.159/(635.0*kappa^2 + 1.0)^(1/2) - 1.0*(atan(0.159/(635.0*kappa^2 + 1.0)^(1/2)) - 0.159/(635.0*kappa^2 + 1.0)^(1/2))*(2.08e-4*Fz + 0.117)))*(((atan(0.159/(635.0*kappa^2 + 1.0)^(1/2)) - 0.159/(635.0*kappa^2 + 1.0)^(1/2))*(2.08e-4*Fz + 0.117) - 0.159/(635.0*kappa^2 + 1.0)^(1/2))^2 + 1.0)) + (0.989*cos(0.989*atan((atan(0.159/(635.0*kappa^2 + 1.0)^(1/2)) - 0.159/(635.0*kappa^2 + 1.0)^(1/2))*(2.08e-4*Fz + 0.117) - 0.159/(635.0*kappa^2 + 1.0)^(1/2)))*sin(0.989*atan(0.159/(635.0*kappa^2 + 1.0)^(1/2) - 1.0*(atan(0.159/(635.0*kappa^2 + 1.0)^(1/2)) - 0.159/(635.0*kappa^2 + 1.0)^(1/2))*(2.08e-4*Fz + 0.117)))*(1.0e-4*Fz^2*LMU - 1.92*Fz*LMU*sin(1.41*atan((4.17e-5*Fz - 0.46)*(0.524*sign(kappa - 1.57e-6*Fz + 6.66e-4) + 1.0)*(atan((0.7*Fz*exp(0.0135 - 1.35e-5*Fz)*(0.015*Fz + 67.7)*(kappa - 1.57e-6*Fz + 6.66e-4))/(2.71*Fz*LMU + 0.01)) - (0.7*Fz*exp(0.0135 - 1.35e-5*Fz)*(0.015*Fz + 67.7)*(kappa - 1.57e-6*Fz + 6.66e-4))/(2.71*Fz*LMU + 0.01)) - (0.7*Fz*exp(0.0135 - 1.35e-5*Fz)*(0.015*Fz + 67.7)*(kappa - 1.57e-6*Fz + 6.66e-4))/(2.71*Fz*LMU + 0.01))))*((2.08e-4*Fz + 0.117)*((101.0*kappa)/(635.0*kappa^2 + 1.0)^(3/2) - (101.0*kappa)/((635.0*kappa^2 + 1.0)^(3/2)*(0.0253/(635.0*kappa^2 + 1.0) + 1.0))) + (101.0*kappa)/(635.0*kappa^2 + 1.0)^(3/2))*(rs^2/Iw - 0.0148*kappa + 0.0148))/(vx*cos(0.989*atan(0.159/(635.0*kappa^2 + 1.0)^(1/2) - 1.0*(atan(0.159/(635.0*kappa^2 + 1.0)^(1/2)) - 0.159/(635.0*kappa^2 + 1.0)^(1/2))*(2.08e-4*Fz + 0.117)))^2*((1.0*(atan(0.159/(635.0*kappa^2 + 1.0)^(1/2)) - 0.159/(635.0*kappa^2 + 1.0)^(1/2))*(2.08e-4*Fz + 0.117) - 0.159/(635.0*kappa^2 + 1.0)^(1/2))^2 + 1.0)) - (2.71*Fz*LMU*cos(1.41*atan((4.17e-5*Fz - 0.46)*(0.524*sign(kappa - 1.57e-6*Fz + 6.66e-4) + 1.0)*(atan((0.7*Fz*exp(0.0135 - 1.35e-5*Fz)*(0.015*Fz + 67.7)*(kappa - 1.57e-6*Fz + 6.66e-4))/(2.71*Fz*LMU + 0.01)) - (0.7*Fz*exp(0.0135 - 1.35e-5*Fz)*(0.015*Fz + 67.7)*(kappa - 1.57e-6*Fz + 6.66e-4))/(2.71*Fz*LMU + 0.01)) - (0.7*Fz*exp(0.0135 - 1.35e-5*Fz)*(0.015*Fz + 67.7)*(kappa - 1.57e-6*Fz + 6.66e-4))/(2.71*Fz*LMU + 0.01)))*cos(0.989*atan((atan(0.159/(635.0*kappa^2 + 1.0)^(1/2)) - 0.159/(635.0*kappa^2 + 1.0)^(1/2))*(2.08e-4*Fz + 0.117) - 0.159/(635.0*kappa^2 + 1.0)^(1/2)))*(((0.7*Fz*exp(0.0135 - 1.35e-5*Fz)*(0.015*Fz + 67.7))/(2.71*Fz*LMU + 0.01) - (0.7*Fz*exp(0.0135 - 1.35e-5*Fz)*(0.015*Fz + 67.7))/(((0.49*Fz^2*exp(0.027 - 2.7e-5*Fz)*(0.015*Fz + 67.7)^2*(kappa - 1.57e-6*Fz + 6.66e-4)^2)/(2.71*Fz*LMU + 0.01)^2 + 1.0)*(2.71*Fz*LMU + 0.01)))*(4.17e-5*Fz - 0.46)*(0.524*sign(kappa - 1.57e-6*Fz + 6.66e-4) + 1.0) - 1.05*dirac(kappa - 1.57e-6*Fz + 6.66e-4)*(4.17e-5*Fz - 0.46)*(atan((0.7*Fz*exp(0.0135 - 1.35e-5*Fz)*(0.015*Fz + 67.7)*(kappa - 1.57e-6*Fz + 6.66e-4))/(2.71*Fz*LMU + 0.01)) - (0.7*Fz*exp(0.0135 - 1.35e-5*Fz)*(0.015*Fz + 67.7)*(kappa - 1.57e-6*Fz + 6.66e-4))/(2.71*Fz*LMU + 0.01)) + (0.7*Fz*exp(0.0135 - 1.35e-5*Fz)*(0.015*Fz + 67.7))/(2.71*Fz*LMU + 0.01))*(rs^2/Iw - 0.0148*kappa + 0.0148))/(vx*cos(0.989*atan(0.159/(635.0*kappa^2 + 1.0)^(1/2) - 1.0*(atan(0.159/(635.0*kappa^2 + 1.0)^(1/2)) - 0.159/(635.0*kappa^2 + 1.0)^(1/2))*(2.08e-4*Fz + 0.117)))*(((4.17e-5*Fz - 0.46)*(0.524*sign(kappa - 1.57e-6*Fz + 6.66e-4) + 1.0)*(atan((0.7*Fz*exp(0.0135 - 1.35e-5*Fz)*(0.015*Fz + 67.7)*(kappa - 1.57e-6*Fz + 6.66e-4))/(2.71*Fz*LMU + 0.01)) - (0.7*Fz*exp(0.0135 - 1.35e-5*Fz)*(0.015*Fz + 67.7)*(kappa - 1.57e-6*Fz + 6.66e-4))/(2.71*Fz*LMU + 0.01)) - (0.7*Fz*exp(0.0135 - 1.35e-5*Fz)*(0.015*Fz + 67.7)*(kappa - 1.57e-6*Fz + 6.66e-4))/(2.71*Fz*LMU + 0.01))^2 + 1.0))

LMU = 0.8;
rs = 0.235;
Iw = 2e5/1e6;
dt = 0.2;
tau = 13.5;
dt = 0.02;
g = 9.81;

B = rs^2/Iw/vx*dt;

fx = -(1.0*cos(0.989*atan((atan(0.159/(635.0*kappa^2 + 1.0)^(1/2)) - 0.159/(635.0*kappa^2 + 1.0)^(1/2))*(2.08e-4*Fz + 0.117) - 0.159/(635.0*kappa^2 + 1.0)^(1/2)))*(1.0e-4*Fz^2*LMU - 1.92*Fz*LMU*sin(1.41*atan((4.17e-5*Fz - 0.46)*(0.524*sign(kappa - 1.57e-6*Fz + 6.66e-4) + 1.0)*(atan((0.7*Fz*exp(0.0135 - 1.35e-5*Fz)*(0.015*Fz + 67.7)*(kappa - 1.57e-6*Fz + 6.66e-4))/(2.71*Fz*LMU + 0.01)) - (0.7*Fz*exp(0.0135 - 1.35e-5*Fz)*(0.015*Fz + 67.7)*(kappa - 1.57e-6*Fz + 6.66e-4))/(2.71*Fz*LMU + 0.01)) - (0.7*Fz*exp(0.0135 - 1.35e-5*Fz)*(0.015*Fz + 67.7)*(kappa - 1.57e-6*Fz + 6.66e-4))/(2.71*Fz*LMU + 0.01))))*(rs^2/Iw - 0.0148*kappa + 0.0148))/(vx*cos(0.989*atan((atan(0.159/(635.0*kappa^2 + 1.0)^(1/2)) - 0.159/(635.0*kappa^2 + 1.0)^(1/2))*(2.08e-4*Fz + 0.117) - 0.159/(635.0*kappa^2 + 1.0)^(1/2))));
delta_kappa = 0.001;
kappa_plus = kappa + delta_kappa;
fx_plus = -(1.0*cos(0.989*atan((atan(0.159/(635.0*kappa_plus^2 + 1.0)^(1/2)) - 0.159/(635.0*kappa_plus^2 + 1.0)^(1/2))*(2.08e-4*Fz + 0.117) - 0.159/(635.0*kappa_plus^2 + 1.0)^(1/2)))*(1.0e-4*Fz^2*LMU - 1.92*Fz*LMU*sin(1.41*atan((4.17e-5*Fz - 0.46)*(0.524*sign(kappa_plus - 1.57e-6*Fz + 6.66e-4) + 1.0)*(atan((0.7*Fz*exp(0.0135 - 1.35e-5*Fz)*(0.015*Fz + 67.7)*(kappa_plus - 1.57e-6*Fz + 6.66e-4))/(2.71*Fz*LMU + 0.01)) - (0.7*Fz*exp(0.0135 - 1.35e-5*Fz)*(0.015*Fz + 67.7)*(kappa_plus - 1.57e-6*Fz + 6.66e-4))/(2.71*Fz*LMU + 0.01)) - (0.7*Fz*exp(0.0135 - 1.35e-5*Fz)*(0.015*Fz + 67.7)*(kappa_plus - 1.57e-6*Fz + 6.66e-4))/(2.71*Fz*LMU + 0.01))))*(rs^2/Iw - 0.0148*kappa_plus + 0.0148))/(vx*cos(0.989*atan((atan(0.159/(635.0*kappa_plus^2 + 1.0)^(1/2)) - 0.159/(635.0*kappa_plus^2 + 1.0)^(1/2))*(2.08e-4*Fz + 0.117) - 0.159/(635.0*kappa_plus^2 + 1.0)^(1/2))));

Astar = (fx_plus - fx)/delta_kappa;

A = (1 + Astar*dt);

% ~~~~~~~~~~~~~~~~~~~~~~~~~~~~~~~~~~~~~~~~~~~~~~~~~~~~~~~~~~~~~~~~~~~~~~~ %
kappa_ref = 0.1;

% Q = 1e6;
Q = 1e3;
R = 0e-5;

u = u_max_old + (B*Q*B + R)*( (Q*B)*kappa_ref - (A*Q*B)*kappa )/tau;
end

== matlab function TVModel_Simulation_21/Subsystem/Subsystem1/Slip Control/Traction Control/Subsystem2/MATLAB Function3 ==
  data: u_max_old input; vx input; u output; Fz input; kappa input
function u = linear_mpc(u_max_old,vx,Fz,kappa)

% Astar = (0.0148*cos(0.989*atan((atan(0.159/(635.0*kappa^2 + 1.0)^(1/2)) - 0.159/(635.0*kappa^2 + 1.0)^(1/2))*(2.08e-4*Fz + 0.117) - 0.159/(635.0*kappa^2 + 1.0)^(1/2)))*(1.0e-4*Fz^2*LMU - 1.92*Fz*LMU*sin(1.41*atan((4.17e-5*Fz - 0.46)*(0.524*sign(kappa - 1.57e-6*Fz + 6.66e-4) + 1.0)*(atan((0.7*Fz*exp(0.0135 - 1.35e-5*Fz)*(0.015*Fz + 67.7)*(kappa - 1.57e-6*Fz + 6.66e-4))/(2.71*Fz*LMU + 0.01)) - (0.7*Fz*exp(0.0135 - 1.35e-5*Fz)*(0.015*Fz + 67.7)*(kappa - 1.57e-6*Fz + 6.66e-4))/(2.71*Fz*LMU + 0.01)) - (0.7*Fz*exp(0.0135 - 1.35e-5*Fz)*(0.015*Fz + 67.7)*(kappa - 1.57e-6*Fz + 6.66e-4))/(2.71*Fz*LMU + 0.01)))))/(vx*cos(0.989*atan(0.159/(635.0*kappa^2 + 1.0)^(1/2) - 1.0*(atan(0.159/(635.0*kappa^2 + 1.0)^(1/2)) - 0.159/(635.0*kappa^2 + 1.0)^(1/2))*(2.08e-4*Fz + 0.117)))) + (0.989*sin(0.989*atan((atan(0.159/(635.0*kappa^2 + 1.0)^(1/2)) - 0.159/(635.0*kappa^2 + 1.0)^(1/2))*(2.08e-4*Fz + 0.117) - 0.159/(635.0*kappa^2 + 1.0)^(1/2)))*(1.0e-4*Fz^2*LMU - 1.92*Fz*LMU*sin(1.41*atan((4.17e-5*Fz - 0.46)*(0.524*sign(kappa - 1.57e-6*Fz + 6.66e-4) + 1.0)*(atan((0.7*Fz*exp(0.0135 - 1.35e-5*Fz)*(0.015*Fz + 67.7)*(kappa - 1.57e-6*Fz + 6.66e-4))/(2.71*Fz*LMU + 0.01)) - (0.7*Fz*exp(0.0135 - 1.35e-5*Fz)*(0.015*Fz + 67.7)*(kappa - 1.57e-6*Fz + 6.66e-4))/(2.71*Fz*LMU + 0.01)) - (0.7*Fz*exp(0.0135 - 1.35e-5*Fz)*(0.015*Fz + 67.7)*(kappa - 1.57e-6*Fz + 6.66e-4))/(2.71*Fz*LMU + 0.01))))*((2.08e-4*Fz + 0.117)*((101.0*kappa)/(635.0*kappa^2 + 1.0)^(3/2) - (101.0*kappa)/((635.0*kappa^2 + 1.0)^(3/2)*(0.0254/(635.0*kappa^2 + 1.0) + 1.0))) + (101.0*kappa)/(635.0*kappa^2 + 1.0)^(3/2))*(rs^2/Iw - 0.0148*kappa + 0.0148))/(vx*cos(0.989*atan(0.159/(635.0*kappa^2 + 1.0)^(1/2) - 1.0*(atan(0.159/(635.0*kappa^2 + 1.0)^(1/2)) - 0.159/(635.0*kappa^2 + 1.0)^(1/2))*(2.08e-4*Fz + 0.117)))*(((atan(0.159/(635.0*kappa^2 + 1.0)^(1/2)) - 0.159/(635.0*kappa^2 + 1.0)^(1/2))*(2.08e-4*Fz + 0.117) - 0.159/(635.0*kappa^2 + 1.0)^(1/2))^2 + 1.0)) + (0.989*cos(0.989*atan((atan(0.159/(635.0*kappa^2 + 1.0)^(1/2)) - 0.159/(635.0*kappa^2 + 1.0)^(1/2))*(2.08e-4*Fz + 0.117) - 0.159/(635.0*kappa^2 + 1.0)^(1/2)))*sin(0.989*atan(0.159/(635.0*kappa^2 + 1.0)^(1/2) - 1.0*(atan(0.159/(635.0*kappa^2 + 1.0)^(1/2)) - 0.159/(635.0*kappa^2 + 1.0)^(1/2))*(2.08e-4*Fz + 0.117)))*(1.0e-4*Fz^2*LMU - 1.92*Fz*LMU*sin(1.41*atan((4.17e-5*Fz - 0.46)*(0.524*sign(kappa - 1.57e-6*Fz + 6.66e-4) + 1.0)*(atan((0.7*Fz*exp(0.0135 - 1.35e-5*Fz)*(0.015*Fz + 67.7)*(kappa - 1.57e-6*Fz + 6.66e-4))/(2.71*Fz*LMU + 0.01)) - (0.7*Fz*exp(0.0135 - 1.35e-5*Fz)*(0.015*Fz + 67.7)*(kappa - 1.57e-6*Fz + 6.66e-4))/(2.71*Fz*LMU + 0.01)) - (0.7*Fz*exp(0.0135 - 1.35e-5*Fz)*(0.015*Fz + 67.7)*(kappa - 1.57e-6*Fz + 6.66e-4))/(2.71*Fz*LMU + 0.01))))*((2.08e-4*Fz + 0.117)*((101.0*kappa)/(635.0*kappa^2 + 1.0)^(3/2) - (101.0*kappa)/((635.0*kappa^2 + 1.0)^(3/2)*(0.0253/(635.0*kappa^2 + 1.0) + 1.0))) + (101.0*kappa)/(635.0*kappa^2 + 1.0)^(3/2))*(rs^2/Iw - 0.0148*kappa + 0.0148))/(vx*cos(0.989*atan(0.159/(635.0*kappa^2 + 1.0)^(1/2) - 1.0*(atan(0.159/(635.0*kappa^2 + 1.0)^(1/2)) - 0.159/(635.0*kappa^2 + 1.0)^(1/2))*(2.08e-4*Fz + 0.117)))^2*((1.0*(atan(0.159/(635.0*kappa^2 + 1.0)^(1/2)) - 0.159/(635.0*kappa^2 + 1.0)^(1/2))*(2.08e-4*Fz + 0.117) - 0.159/(635.0*kappa^2 + 1.0)^(1/2))^2 + 1.0)) - (2.71*Fz*LMU*cos(1.41*atan((4.17e-5*Fz - 0.46)*(0.524*sign(kappa - 1.57e-6*Fz + 6.66e-4) + 1.0)*(atan((0.7*Fz*exp(0.0135 - 1.35e-5*Fz)*(0.015*Fz + 67.7)*(kappa - 1.57e-6*Fz + 6.66e-4))/(2.71*Fz*LMU + 0.01)) - (0.7*Fz*exp(0.0135 - 1.35e-5*Fz)*(0.015*Fz + 67.7)*(kappa - 1.57e-6*Fz + 6.66e-4))/(2.71*Fz*LMU + 0.01)) - (0.7*Fz*exp(0.0135 - 1.35e-5*Fz)*(0.015*Fz + 67.7)*(kappa - 1.57e-6*Fz + 6.66e-4))/(2.71*Fz*LMU + 0.01)))*cos(0.989*atan((atan(0.159/(635.0*kappa^2 + 1.0)^(1/2)) - 0.159/(635.0*kappa^2 + 1.0)^(1/2))*(2.08e-4*Fz + 0.117) - 0.159/(635.0*kappa^2 + 1.0)^(1/2)))*(((0.7*Fz*exp(0.0135 - 1.35e-5*Fz)*(0.015*Fz + 67.7))/(2.71*Fz*LMU + 0.01) - (0.7*Fz*exp(0.0135 - 1.35e-5*Fz)*(0.015*Fz + 67.7))/(((0.49*Fz^2*exp(0.027 - 2.7e-5*Fz)*(0.015*Fz + 67.7)^2*(kappa - 1.57e-6*Fz + 6.66e-4)^2)/(2.71*Fz*LMU + 0.01)^2 + 1.0)*(2.71*Fz*LMU + 0.01)))*(4.17e-5*Fz - 0.46)*(0.524*sign(kappa - 1.57e-6*Fz + 6.66e-4) + 1.0) - 1.05*dirac(kappa - 1.57e-6*Fz + 6.66e-4)*(4.17e-5*Fz - 0.46)*(atan((0.7*Fz*exp(0.0135 - 1.35e-5*Fz)*(0.015*Fz + 67.7)*(kappa - 1.57e-6*Fz + 6.66e-4))/(2.71*Fz*LMU + 0.01)) - (0.7*Fz*exp(0.0135 - 1.35e-5*Fz)*(0.015*Fz + 67.7)*(kappa - 1.57e-6*Fz + 6.66e-4))/(2.71*Fz*LMU + 0.01)) + (0.7*Fz*exp(0.0135 - 1.35e-5*Fz)*(0.015*Fz + 67.7))/(2.71*Fz*LMU + 0.01))*(rs^2/Iw - 0.0148*kappa + 0.0148))/(vx*cos(0.989*atan(0.159/(635.0*kappa^2 + 1.0)^(1/2) - 1.0*(atan(0.159/(635.0*kappa^2 + 1.0)^(1/2)) - 0.159/(635.0*kappa^2 + 1.0)^(1/2))*(2.08e-4*Fz + 0.117)))*(((4.17e-5*Fz - 0.46)*(0.524*sign(kappa - 1.57e-6*Fz + 6.66e-4) + 1.0)*(atan((0.7*Fz*exp(0.0135 - 1.35e-5*Fz)*(0.015*Fz + 67.7)*(kappa - 1.57e-6*Fz + 6.66e-4))/(2.71*Fz*LMU + 0.01)) - (0.7*Fz*exp(0.0135 - 1.35e-5*Fz)*(0.015*Fz + 67.7)*(kappa - 1.57e-6*Fz + 6.66e-4))/(2.71*Fz*LMU + 0.01)) - (0.7*Fz*exp(0.0135 - 1.35e-5*Fz)*(0.015*Fz + 67.7)*(kappa - 1.57e-6*Fz + 6.66e-4))/(2.71*Fz*LMU + 0.01))^2 + 1.0))

LMU = 0.8;
rs = 0.235;
Iw = 2e5/1e6;
dt = 0.2;
tau = 13.5;
dt = 0.02;
g = 9.81;

B = rs^2/Iw/vx*dt;

fx = -(1.0*cos(0.989*atan((atan(0.159/(635.0*kappa^2 + 1.0)^(1/2)) - 0.159/(635.0*kappa^2 + 1.0)^(1/2))*(2.08e-4*Fz + 0.117) - 0.159/(635.0*kappa^2 + 1.0)^(1/2)))*(1.0e-4*Fz^2*LMU - 1.92*Fz*LMU*sin(1.41*atan((4.17e-5*Fz - 0.46)*(0.524*sign(kappa - 1.57e-6*Fz + 6.66e-4) + 1.0)*(atan((0.7*Fz*exp(0.0135 - 1.35e-5*Fz)*(0.015*Fz + 67.7)*(kappa - 1.57e-6*Fz + 6.66e-4))/(2.71*Fz*LMU + 0.01)) - (0.7*Fz*exp(0.0135 - 1.35e-5*Fz)*(0.015*Fz + 67.7)*(kappa - 1.57e-6*Fz + 6.66e-4))/(2.71*Fz*LMU + 0.01)) - (0.7*Fz*exp(0.0135 - 1.35e-5*Fz)*(0.015*Fz + 67.7)*(kappa - 1.57e-6*Fz + 6.66e-4))/(2.71*Fz*LMU + 0.01))))*(rs^2/Iw - 0.0148*kappa + 0.0148))/(vx*cos(0.989*atan((atan(0.159/(635.0*kappa^2 + 1.0)^(1/2)) - 0.159/(635.0*kappa^2 + 1.0)^(1/2))*(2.08e-4*Fz + 0.117) - 0.159/(635.0*kappa^2 + 1.0)^(1/2))));
delta_kappa = 0.001;
kappa_plus = kappa + delta_kappa;
fx_plus = -(1.0*cos(0.989*atan((atan(0.159/(635.0*kappa_plus^2 + 1.0)^(1/2)) - 0.159/(635.0*kappa_plus^2 + 1.0)^(1/2))*(2.08e-4*Fz + 0.117) - 0.159/(635.0*kappa_plus^2 + 1.0)^(1/2)))*(1.0e-4*Fz^2*LMU - 1.92*Fz*LMU*sin(1.41*atan((4.17e-5*Fz - 0.46)*(0.524*sign(kappa_plus - 1.57e-6*Fz + 6.66e-4) + 1.0)*(atan((0.7*Fz*exp(0.0135 - 1.35e-5*Fz)*(0.015*Fz + 67.7)*(kappa_plus - 1.57e-6*Fz + 6.66e-4))/(2.71*Fz*LMU + 0.01)) - (0.7*Fz*exp(0.0135 - 1.35e-5*Fz)*(0.015*Fz + 67.7)*(kappa_plus - 1.57e-6*Fz + 6.66e-4))/(2.71*Fz*LMU + 0.01)) - (0.7*Fz*exp(0.0135 - 1.35e-5*Fz)*(0.015*Fz + 67.7)*(kappa_plus - 1.57e-6*Fz + 6.66e-4))/(2.71*Fz*LMU + 0.01))))*(rs^2/Iw - 0.0148*kappa_plus + 0.0148))/(vx*cos(0.989*atan((atan(0.159/(635.0*kappa_plus^2 + 1.0)^(1/2)) - 0.159/(635.0*kappa_plus^2 + 1.0)^(1/2))*(2.08e-4*Fz + 0.117) - 0.159/(635.0*kappa_plus^2 + 1.0)^(1/2))));

Astar = (fx_plus - fx)/delta_kappa;

A = (1 + Astar*dt);

% ~~~~~~~~~~~~~~~~~~~~~~~~~~~~~~~~~~~~~~~~~~~~~~~~~~~~~~~~~~~~~~~~~~~~~~~ %
kappa_ref = 0.1;

% Q = 1e6;
Q = 1e3
R = 0e-5;

u = u_max_old + (B*Q*B + R)*( (Q*B)*kappa_ref - (A*Q*B)*kappa )/tau;
end

== matlab function TVModel_Simulation_21/Subsystem/Subsystem1/Slip Control/Traction Control/Subsystem2/MATLAB Function4 ==
  data: u_max_old input; vx input; u output; Fz input; kappa input
function u = linear_mpc(u_max_old,vx,Fz,kappa)

% Astar = (0.0148*cos(0.989*atan((atan(0.159/(635.0*kappa^2 + 1.0)^(1/2)) - 0.159/(635.0*kappa^2 + 1.0)^(1/2))*(2.08e-4*Fz + 0.117) - 0.159/(635.0*kappa^2 + 1.0)^(1/2)))*(1.0e-4*Fz^2*LMU - 1.92*Fz*LMU*sin(1.41*atan((4.17e-5*Fz - 0.46)*(0.524*sign(kappa - 1.57e-6*Fz + 6.66e-4) + 1.0)*(atan((0.7*Fz*exp(0.0135 - 1.35e-5*Fz)*(0.015*Fz + 67.7)*(kappa - 1.57e-6*Fz + 6.66e-4))/(2.71*Fz*LMU + 0.01)) - (0.7*Fz*exp(0.0135 - 1.35e-5*Fz)*(0.015*Fz + 67.7)*(kappa - 1.57e-6*Fz + 6.66e-4))/(2.71*Fz*LMU + 0.01)) - (0.7*Fz*exp(0.0135 - 1.35e-5*Fz)*(0.015*Fz + 67.7)*(kappa - 1.57e-6*Fz + 6.66e-4))/(2.71*Fz*LMU + 0.01)))))/(vx*cos(0.989*atan(0.159/(635.0*kappa^2 + 1.0)^(1/2) - 1.0*(atan(0.159/(635.0*kappa^2 + 1.0)^(1/2)) - 0.159/(635.0*kappa^2 + 1.0)^(1/2))*(2.08e-4*Fz + 0.117)))) + (0.989*sin(0.989*atan((atan(0.159/(635.0*kappa^2 + 1.0)^(1/2)) - 0.159/(635.0*kappa^2 + 1.0)^(1/2))*(2.08e-4*Fz + 0.117) - 0.159/(635.0*kappa^2 + 1.0)^(1/2)))*(1.0e-4*Fz^2*LMU - 1.92*Fz*LMU*sin(1.41*atan((4.17e-5*Fz - 0.46)*(0.524*sign(kappa - 1.57e-6*Fz + 6.66e-4) + 1.0)*(atan((0.7*Fz*exp(0.0135 - 1.35e-5*Fz)*(0.015*Fz + 67.7)*(kappa - 1.57e-6*Fz + 6.66e-4))/(2.71*Fz*LMU + 0.01)) - (0.7*Fz*exp(0.0135 - 1.35e-5*Fz)*(0.015*Fz + 67.7)*(kappa - 1.57e-6*Fz + 6.66e-4))/(2.71*Fz*LMU + 0.01)) - (0.7*Fz*exp(0.0135 - 1.35e-5*Fz)*(0.015*Fz + 67.7)*(kappa - 1.57e-6*Fz + 6.66e-4))/(2.71*Fz*LMU + 0.01))))*((2.08e-4*Fz + 0.117)*((101.0*kappa)/(635.0*kappa^2 + 1.0)^(3/2) - (101.0*kappa)/((635.0*kappa^2 + 1.0)^(3/2)*(0.0254/(635.0*kappa^2 + 1.0) + 1.0))) + (101.0*kappa)/(635.0*kappa^2 + 1.0)^(3/2))*(rs^2/Iw - 0.0148*kappa + 0.0148))/(vx*cos(0.989*atan(0.159/(635.0*kappa^2 + 1.0)^(1/2) - 1.0*(atan(0.159/(635.0*kappa^2 + 1.0)^(1/2)) - 0.159/(635.0*kappa^2 + 1.0)^(1/2))*(2.08e-4*Fz + 0.117)))*(((atan(0.159/(635.0*kappa^2 + 1.0)^(1/2)) - 0.159/(635.0*kappa^2 + 1.0)^(1/2))*(2.08e-4*Fz + 0.117) - 0.159/(635.0*kappa^2 + 1.0)^(1/2))^2 + 1.0)) + (0.989*cos(0.989*atan((atan(0.159/(635.0*kappa^2 + 1.0)^(1/2)) - 0.159/(635.0*kappa^2 + 1.0)^(1/2))*(2.08e-4*Fz + 0.117) - 0.159/(635.0*kappa^2 + 1.0)^(1/2)))*sin(0.989*atan(0.159/(635.0*kappa^2 + 1.0)^(1/2) - 1.0*(atan(0.159/(635.0*kappa^2 + 1.0)^(1/2)) - 0.159/(635.0*kappa^2 + 1.0)^(1/2))*(2.08e-4*Fz + 0.117)))*(1.0e-4*Fz^2*LMU - 1.92*Fz*LMU*sin(1.41*atan((4.17e-5*Fz - 0.46)*(0.524*sign(kappa - 1.57e-6*Fz + 6.66e-4) + 1.0)*(atan((0.7*Fz*exp(0.0135 - 1.35e-5*Fz)*(0.015*Fz + 67.7)*(kappa - 1.57e-6*Fz + 6.66e-4))/(2.71*Fz*LMU + 0.01)) - (0.7*Fz*exp(0.0135 - 1.35e-5*Fz)*(0.015*Fz + 67.7)*(kappa - 1.57e-6*Fz + 6.66e-4))/(2.71*Fz*LMU + 0.01)) - (0.7*Fz*exp(0.0135 - 1.35e-5*Fz)*(0.015*Fz + 67.7)*(kappa - 1.57e-6*Fz + 6.66e-4))/(2.71*Fz*LMU + 0.01))))*((2.08e-4*Fz + 0.117)*((101.0*kappa)/(635.0*kappa^2 + 1.0)^(3/2) - (101.0*kappa)/((635.0*kappa^2 + 1.0)^(3/2)*(0.0253/(635.0*kappa^2 + 1.0) + 1.0))) + (101.0*kappa)/(635.0*kappa^2 + 1.0)^(3/2))*(rs^2/Iw - 0.0148*kappa + 0.0148))/(vx*cos(0.989*atan(0.159/(635.0*kappa^2 + 1.0)^(1/2) - 1.0*(atan(0.159/(635.0*kappa^2 + 1.0)^(1/2)) - 0.159/(635.0*kappa^2 + 1.0)^(1/2))*(2.08e-4*Fz + 0.117)))^2*((1.0*(atan(0.159/(635.0*kappa^2 + 1.0)^(1/2)) - 0.159/(635.0*kappa^2 + 1.0)^(1/2))*(2.08e-4*Fz + 0.117) - 0.159/(635.0*kappa^2 + 1.0)^(1/2))^2 + 1.0)) - (2.71*Fz*LMU*cos(1.41*atan((4.17e-5*Fz - 0.46)*(0.524*sign(kappa - 1.57e-6*Fz + 6.66e-4) + 1.0)*(atan((0.7*Fz*exp(0.0135 - 1.35e-5*Fz)*(0.015*Fz + 67.7)*(kappa - 1.57e-6*Fz + 6.66e-4))/(2.71*Fz*LMU + 0.01)) - (0.7*Fz*exp(0.0135 - 1.35e-5*Fz)*(0.015*Fz + 67.7)*(kappa - 1.57e-6*Fz + 6.66e-4))/(2.71*Fz*LMU + 0.01)) - (0.7*Fz*exp(0.0135 - 1.35e-5*Fz)*(0.015*Fz + 67.7)*(kappa - 1.57e-6*Fz + 6.66e-4))/(2.71*Fz*LMU + 0.01)))*cos(0.989*atan((atan(0.159/(635.0*kappa^2 + 1.0)^(1/2)) - 0.159/(635.0*kappa^2 + 1.0)^(1/2))*(2.08e-4*Fz + 0.117) - 0.159/(635.0*kappa^2 + 1.0)^(1/2)))*(((0.7*Fz*exp(0.0135 - 1.35e-5*Fz)*(0.015*Fz + 67.7))/(2.71*Fz*LMU + 0.01) - (0.7*Fz*exp(0.0135 - 1.35e-5*Fz)*(0.015*Fz + 67.7))/(((0.49*Fz^2*exp(0.027 - 2.7e-5*Fz)*(0.015*Fz + 67.7)^2*(kappa - 1.57e-6*Fz + 6.66e-4)^2)/(2.71*Fz*LMU + 0.01)^2 + 1.0)*(2.71*Fz*LMU + 0.01)))*(4.17e-5*Fz - 0.46)*(0.524*sign(kappa - 1.57e-6*Fz + 6.66e-4) + 1.0) - 1.05*dirac(kappa - 1.57e-6*Fz + 6.66e-4)*(4.17e-5*Fz - 0.46)*(atan((0.7*Fz*exp(0.0135 - 1.35e-5*Fz)*(0.015*Fz + 67.7)*(kappa - 1.57e-6*Fz + 6.66e-4))/(2.71*Fz*LMU + 0.01)) - (0.7*Fz*exp(0.0135 - 1.35e-5*Fz)*(0.015*Fz + 67.7)*(kappa - 1.57e-6*Fz + 6.66e-4))/(2.71*Fz*LMU + 0.01)) + (0.7*Fz*exp(0.0135 - 1.35e-5*Fz)*(0.015*Fz + 67.7))/(2.71*Fz*LMU + 0.01))*(rs^2/Iw - 0.0148*kappa + 0.0148))/(vx*cos(0.989*atan(0.159/(635.0*kappa^2 + 1.0)^(1/2) - 1.0*(atan(0.159/(635.0*kappa^2 + 1.0)^(1/2)) - 0.159/(635.0*kappa^2 + 1.0)^(1/2))*(2.08e-4*Fz + 0.117)))*(((4.17e-5*Fz - 0.46)*(0.524*sign(kappa - 1.57e-6*Fz + 6.66e-4) + 1.0)*(atan((0.7*Fz*exp(0.0135 - 1.35e-5*Fz)*(0.015*Fz + 67.7)*(kappa - 1.57e-6*Fz + 6.66e-4))/(2.71*Fz*LMU + 0.01)) - (0.7*Fz*exp(0.0135 - 1.35e-5*Fz)*(0.015*Fz + 67.7)*(kappa - 1.57e-6*Fz + 6.66e-4))/(2.71*Fz*LMU + 0.01)) - (0.7*Fz*exp(0.0135 - 1.35e-5*Fz)*(0.015*Fz + 67.7)*(kappa - 1.57e-6*Fz + 6.66e-4))/(2.71*Fz*LMU + 0.01))^2 + 1.0))

LMU = 0.8;
rs = 0.235;
Iw = 2e5/1e6;
dt = 0.2;
tau = 13.5;
dt = 0.02;
g = 9.81;

B = rs^2/Iw/vx*dt;

fx = -(1.0*cos(0.989*atan((atan(0.159/(635.0*kappa^2 + 1.0)^(1/2)) - 0.159/(635.0*kappa^2 + 1.0)^(1/2))*(2.08e-4*Fz + 0.117) - 0.159/(635.0*kappa^2 + 1.0)^(1/2)))*(1.0e-4*Fz^2*LMU - 1.92*Fz*LMU*sin(1.41*atan((4.17e-5*Fz - 0.46)*(0.524*sign(kappa - 1.57e-6*Fz + 6.66e-4) + 1.0)*(atan((0.7*Fz*exp(0.0135 - 1.35e-5*Fz)*(0.015*Fz + 67.7)*(kappa - 1.57e-6*Fz + 6.66e-4))/(2.71*Fz*LMU + 0.01)) - (0.7*Fz*exp(0.0135 - 1.35e-5*Fz)*(0.015*Fz + 67.7)*(kappa - 1.57e-6*Fz + 6.66e-4))/(2.71*Fz*LMU + 0.01)) - (0.7*Fz*exp(0.0135 - 1.35e-5*Fz)*(0.015*Fz + 67.7)*(kappa - 1.57e-6*Fz + 6.66e-4))/(2.71*Fz*LMU + 0.01))))*(rs^2/Iw - 0.0148*kappa + 0.0148))/(vx*cos(0.989*atan((atan(0.159/(635.0*kappa^2 + 1.0)^(1/2)) - 0.159/(635.0*kappa^2 + 1.0)^(1/2))*(2.08e-4*Fz + 0.117) - 0.159/(635.0*kappa^2 + 1.0)^(1/2))));
delta_kappa = 0.001;
kappa_plus = kappa + delta_kappa;
fx_plus = -(1.0*cos(0.989*atan((atan(0.159/(635.0*kappa_plus^2 + 1.0)^(1/2)) - 0.159/(635.0*kappa_plus^2 + 1.0)^(1/2))*(2.08e-4*Fz + 0.117) - 0.159/(635.0*kappa_plus^2 + 1.0)^(1/2)))*(1.0e-4*Fz^2*LMU - 1.92*Fz*LMU*sin(1.41*atan((4.17e-5*Fz - 0.46)*(0.524*sign(kappa_plus - 1.57e-6*Fz + 6.66e-4) + 1.0)*(atan((0.7*Fz*exp(0.0135 - 1.35e-5*Fz)*(0.015*Fz + 67.7)*(kappa_plus - 1.57e-6*Fz + 6.66e-4))/(2.71*Fz*LMU + 0.01)) - (0.7*Fz*exp(0.0135 - 1.35e-5*Fz)*(0.015*Fz + 67.7)*(kappa_plus - 1.57e-6*Fz + 6.66e-4))/(2.71*Fz*LMU + 0.01)) - (0.7*Fz*exp(0.0135 - 1.35e-5*Fz)*(0.015*Fz + 67.7)*(kappa_plus - 1.57e-6*Fz + 6.66e-4))/(2.71*Fz*LMU + 0.01))))*(rs^2/Iw - 0.0148*kappa_plus + 0.0148))/(vx*cos(0.989*atan((atan(0.159/(635.0*kappa_plus^2 + 1.0)^(1/2)) - 0.159/(635.0*kappa_plus^2 + 1.0)^(1/2))*(2.08e-4*Fz + 0.117) - 0.159/(635.0*kappa_plus^2 + 1.0)^(1/2))));

Astar = (fx_plus - fx)/delta_kappa;

A = (1 + Astar*dt);

% ~~~~~~~~~~~~~~~~~~~~~~~~~~~~~~~~~~~~~~~~~~~~~~~~~~~~~~~~~~~~~~~~~~~~~~~ %
kappa_ref = 0.1;

% Q = 1e6;
Q = 1e3;
R = 0e-5;

u = u_max_old + (B*Q*B + R)*( (Q*B)*kappa_ref - (A*Q*B)*kappa )/tau;
end

== matlab function TVModel_Simulation_21/Subsystem/Subsystem1/Slip Control/Traction Control/TC/MATLAB Function3 ==
  data: T_old input; T_max output; omega_dot input; alpha input
function T_max = fcn(T_old,omega_dot,alpha)

rs = 0.235;
M = 270/4;
Iw = 2e5/1e6;
tau = 13.5;

T_old = T_old.*tau;

Vw_dot = omega_dot.*rs;
Fd = T_old./rs - Iw.*Vw_dot/(rs^2);

% alpha = 0.9;

T_max = (Iw./(alpha.*M*(rs).^2) + 1).*rs.*Fd;

T_max = T_max./tau;

for i = 1 : length(T_old)
    if T_old(i)/tau < 2
       T_max(i) = 21;
    end
end
